simulink model "shuzitiaoxiang1"  (Simulink 9.2)
settings: Solver=ode45  StartTime=0.0  StopTime=10.0  RelTol=1e-3  EnableMultiTasking=on
libraries: commchan3 x1, dsparch4 x1, commrandsrc2 x1, commsink2 x1, dspsigops x1
settings Model: Creator=Administrator  LastModifiedBy=Administrator
settings DataIOCC: SignalLoggingName=sigsOut
settings OptimizationCC: LifeSpan=auto
settings DebuggingCC: SaveWithParameterizedLinksMsg=none  SignalResolutionControl=TryResolveAllWithWarning  MultiTaskDSMMsg=warning  MultiTaskCondExecSysMsg=none  FcnCallInpInsideContextMsg=error  StateNameClashWarn=none  SFUnexpectedBacktrackingDiag=error  SFNoUnconditionalDefaultTransitionDiag=error  SFExecutionAtInitializationDiag=warning
settings HardwareCC: TargetUnknown=on
settings SFSimCC: SimUseLocalCustomCode=on
settings RTWCC: RTWUseLocalCustomCode=on
settings CodeAppCC: StateflowObjectComments=off
settings GRTTargetCC: TargetLangStandard=C99 (ISO)  GeneratePreprocessorConditionals=Use local settings
settings ConfigComp: CovExternalEMLEnable=on

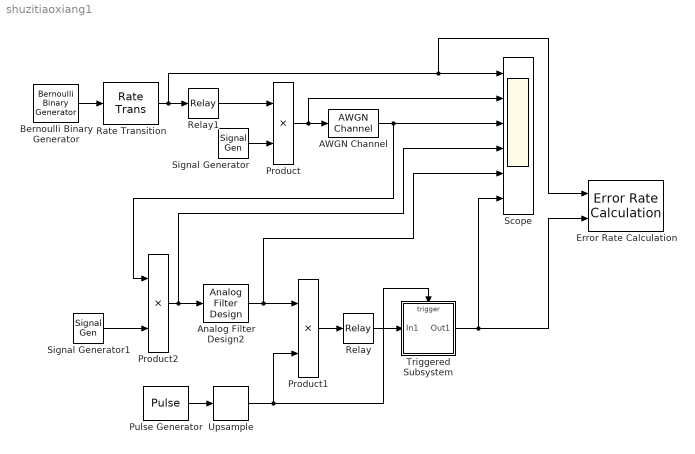
== system shuzitiaoxiang1 ==
  AWGN Channel : commchan3/AWGN Channel  InputProcessing=Columns as channels (frame based)  seed=67  noiseMode=Variance from mask  EbNodB=10  EsNodB=10  SNRdB=10  bitsPerSym=1  Ps=1  Tsym=1  variance=0.5
      settings: SourceProductName=Communications Toolbox
  Analog Filter Design2 : dsparch4/Analog Filter Design  method=Butterworth  filttype=Lowpass  N=2  Wlo=2*pi*3  Whi=80  Rp=2  Rs=40
  Bernoulli Binary Generator : commrandsrc2/Bernoulli Binary Generator  P=0.5  seed=61  Ts=1  frameBased=off  sampPerFrame=1  orient=off  outDataType=double
  Error Rate Calculation : commsink2/Error Rate Calculation  N=0  st_delay=0  cp_mode=Entire frame  subframe=[]  PMode=Workspace  WsName=ErrorVec  RsMode2=off  stop=off  numErr=100  maxBits=1e6
      settings: SourceProductName=Communications Toolbox
  Product : Product  SaturateOnIntegerOverflow=on  OutDataTypeStr=Inherit: Same as first input
  Product1 : Product  SaturateOnIntegerOverflow=on  OutDataTypeStr=Inherit: Same as first input
  Product2 : Product  SaturateOnIntegerOverflow=on  OutDataTypeStr=Inherit: Same as first input
  Pulse Generator : DiscretePulseGenerator  Period=10  PulseWidth=5  SampleTime=0.1
  Rate Transition : RateTransition
  Relay : Relay  OnSwitchValue=0.5  OffSwitchValue=0
  Relay1 : Relay
  Scope : Scope  NumInputPorts=6
  Signal Generator : SignalGenerator  Frequency=2
  Signal Generator1 : SignalGenerator  Frequency=2
  Triggered Subsystem : Subsystem  TreatAsAtomicUnit=on
  Upsample : dspsigops/Upsample  N=10  phase=0  InputProcessing=Columns as channels (frame based)  RateOptions=Allow multirate processing  ic=0  mode=Unused parameter value
  wires:
  Signal Generator/1 -> Product/2
  Bernoulli Binary Generator/1 -> Rate Transition/1
  Product/1 -> AWGN Channel/1, Scope/2
  Product2/1 -> Analog Filter Design2/1, Scope/4
  Pulse Generator/1 -> Upsample/1
  Rate Transition/1 -> Relay1/1, Scope/1, Error Rate Calculation/1
  Relay1/1 -> Product/1
  AWGN Channel/1 -> Scope/3, Product2/1
  Signal Generator1/1 -> Product2/2
  Analog Filter Design2/1 -> Product1/1, Scope/5
  Product1/1 -> Relay/1
  Relay/1 -> Triggered Subsystem/1(In1)
  Upsample/1 -> Triggered Subsystem/Trigger, Product1/2
  Triggered Subsystem/1(Out1) -> Error Rate Calculation/2, Scope/6

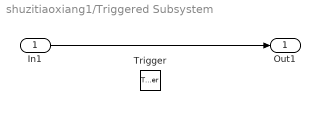
== system shuzitiaoxiang1/Triggered Subsystem ==
  In1 : Inport
  Trigger : TriggerPort  VariantControl=(inherit)
  Out1 : Outport
  wires:
  In1/1 -> Out1/1
